simulink library "NamedStore_lib"  (R2023b)
settings: Solver=VariableStepAuto  StartTime=0.0  StopTime=10.0  RelTol=1e-3
libraries: simulink x1
settings Model: Creator=cbuttril  LastModifiedBy=suvo
settings DataIOCC: SaveFormat=Array  SignalLoggingSaveFormat=ModelDataLogs  ReturnWorkspaceOutputs=off
settings OptimizationCC: BlockReduction=off  BooleanDataType=off
settings DebuggingCC: SaveWithParameterizedLinksMsg=none  UnderspecifiedInitializationDetection=Classic  MergeDetectMultiDrivingBlocksExec=none  SignalResolutionControl=TryResolveAllWithWarning
settings HardwareCC: ProdBitPerPointer=32  ProdBitPerSizeT=32  ProdBitPerPtrDiffT=32  ProdLargestAtomicFloat=None  ProdIntDivRoundTo=Undefined  ProdEndianess=Unspecified  ProdWordSize=32  ProdHWDeviceType=32-bit Generic  TargetUnknown=on
settings ModelReferenceCC: PropagateSignalLabelsOutOfModel=off
settings ConfigComp: CovMetricSettings=dw  CovSaveCumulativeToWorkspaceVar=on  CovSaveSingleToWorkspaceVar=on

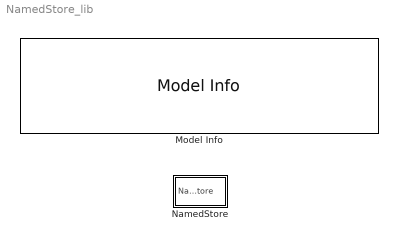
== system NamedStore_lib ==
  Model Info : simulink/Model-Wide Utilities/Model Info  Frame=on  DisplayStringWithTags=|  HorizontalTextAlignment=Center  LeftAlignmentValue=0.5
      | Developed using Matlab Release 2007a
      | 
      | SVN:%<ModelVersion>
      | Last modifed by %<LastModifiedBy> on %<LastModificationDate>
  NamedStore : Subsystem  StopFcn=|  mask(Custom To Workspace Block){Npts=inf, VarName=sout, expand=off}
      | %                                                                                       
      | % script: namedstore_stopfcn                                                            
      | %                                                                                       
      | % Workspace script called by NamedStore block as StopFcn callback.                      
      | %                                                                                       
      | % This converts from fixed name array and  variable list                                
      | % into user names structure.   It also optionally expands fields of the                 
      | % structure  into individual variables.                                                 
      |                                                                                         
      | VarName=get_param(gcb,'VarName');                                                       
      |                                                                                         
      |                                                                                         
      | % If data exists                                                                        
      | if exist(strcat(VarName,'_mat'),'var');                                                 
      |   % Grab field names from diagram                                                       
      |    signal_names=get_param(sprintf('%s/Names',gcb),'InputSignals');                      
      |                                                                                         
      |   % Only works for scalar signals...                                                    
      |   % Doing vectors would require pre-compile of diagram,                                 
      |   % and parsing of "CompliedPortDimensions" parameter.                                  
      |   if length(signal_names) ~=  eval(sprintf('size(%s_mat,2)',VarName));                  
      |     fprintf(1,'Structure ''%s'' not formed, namedsore data remains in matrix form\n',...
      |             VarName);                                                                   
      |     error('NamedStore input contains non-scalar signals');                              
      |   end                                                                                   
      |                                                                                         
      |   % Don't want to augment existing variable                                             
      |   eval(sprintf('clear %s',VarName));                                                    
      |                                                                                         
      |   % Loop through each named variable, assign in structure;                              
      |   for cnt=[1:length(signal_names)],                                                     
      |     eval(sprintf('%s.(signal_names{cnt})=%s_mat(:,cnt);',...                            
      |                  VarName,VarName));                                                     
      |   end                                                                                   
      |                                                                                         
      |                                                                                         
      |                                                                                         
      |   % If selected, expand all fields.                                                     
      |   if (strcmp(get_param(gcb,'expand'),'on' ))                                            
      |     eval(sprintf('expand(%s);',VarName));                                               
      |   end                                                                                   
      |  % Delete tmp name variables from workspace                                             
      |   eval(sprintf('clear %s_mat',VarName));                                                
      |   clear cnt VarName signal_names                                                        
      |  end
      mask prompts: Npts "Limit data points to last"; VarName "Variable Name"; expand "Expand Variables in Base Workspace"
      mask help:
      | Saves simulation data to a workspace variable in a structure format.
      | Input is limited to uniquely named scalar signals.
      | Relies on a stop-fcn callback.
      mask init:
      | set_param(sprintf('%s/To Workspace',gcb),'MaxDataPoints',sprintf('%d',Npts));
      | InSig=get_param(sprintf('%s/Names',gcb),'InputSignals');
      | set_param(sprintf('%s/Names',gcb),'OutputSignals',InSig{1});  % Gotta have one..
      | set_param(sprintf('%s/To Workspace',gcb),'VariableName',strcat(VarName,'_mat'));
      | 
      | 
      | 
      | % Check for duplicates, error out
      | [uni,ndx]=unique(InSig);
      | if length(uni)~=length(InSig),
      |  dups=InSig(setdiff([1:length(InSig)],ndx));
      |  dups
      |  error(sprintf('\nDuplicate signal names in named_store block: %s',dups{:}));
      | end
      mask Display: port_label('input',1,VarName);

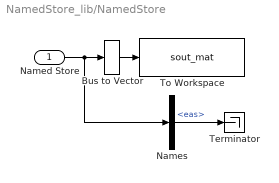
== system NamedStore_lib/NamedStore ==
  Named Store : Inport
  Bus to Vector : BusToVector
  Names : BusSelector  OutputSignals=eas
  Terminator : Terminator
  To Workspace : ToWorkspace  VariableName=sout_mat  SampleTime=-1
      settings: MaxDataPoints=Inf
  wires:
  Bus to Vector/1 -> To Workspace/1
  Names/1 -> Terminator/1  "<eas>"
  Named Store/1 -> Bus to Vector/1, Names/1
